simulink model "LinearInvertedPendulum_closedloop_mc40"  (R2023a)
settings: Solver=FixedStepAuto  StartTime=0.0  StopTime=inf  FixedStep=0.01  RelTol=1e-3  EnableMultiTasking=on
PreLoadFcn:
  | robotParameters;
model workspace (MAT data in the model file):
  axleLength = 0.085
  ticksPerRot = 1200
  wheelR = 0.045
undefined symbols (not defined in the file): DiscIntNeverNeededParam
libraries: M5Core_Library x4, simulink x2, arduinolib x1
settings Model: ExtModeTrigDuration=2  Creator=sseshadr  LastModifiedBy=auw_a
settings SolverCC: AlgebraicLoopSolver=TrustRegion
settings DataIOCC: ReturnWorkspaceOutputs=off
settings OptimizationCC: MaxStackSize=64  EfficientTunableParamExpr=on
settings DebuggingCC: ParameterOverflowMsg=none  ParameterUnderflowMsg=error  ParameterPrecisionLossMsg=none  ParameterTunabilityLossMsg=error  UnconnectedInputMsg=warning  UnconnectedOutputMsg=warning  UnconnectedLineMsg=warning  ArithmeticOperatorsInVariantConditions=warning
settings HardwareCC: ProdBitPerPointer=32  ProdBitPerSizeT=32  ProdBitPerPtrDiffT=32  ProdLargestAtomicInteger=Long  ProdLargestAtomicFloat=Double  ProdWordSize=32  ProdHWDeviceType=ARM Compatible->ARM Cortex
settings ModelReferenceCC: EnableRefExpFcnMdlSchedulingChecks=on
settings SFSimCC: SimUseLocalCustomCode=off  MATLABDynamicMemAlloc=off  CustomCodeUndefinedFunction=UseInterfaceOnly
settings RTWCC: Description=Embedded Coder  SystemTargetFile=ert.tlc  HardwareBoard=ESP32-WROOM(Arduino Compatible)  TLCOptions="-aInlineSetEventsForThisBaseRateFcn=TLC_FALSE -aSuppressMultiTaskScheduler=TLC_FALSE    -aRateBasedStepFcn=0"  TemplateMakefile=ert_default_tmf  GenerateReport=on  RTWUseLocalCustomCode=off  Toolchain=ESP32  BuildConfiguration=Faster Runs  IncludeHyperlinkInReport=on  GenerateTraceInfo=on  GenerateTraceReport=on  GenerateTraceReportSl=on  GenerateTraceReportSf=on  GenerateTraceReportEml=on  DLArmComputeVersion=19.05
settings CodeAppCC: ForceParamTrailComments=on  IgnoreCustomStorageClasses=off  OperatorAnnotations=on  SimulinkDataObjDesc=on  SFDataObjDesc=on  MATLABFcnDesc=on  InsertBlockDesc=on  StateflowObjectComments=on  MATLABSourceComments=on
settings ERTTargetCC: MultiwordLength=2048  SupportContinuousTime=on  SupportVariableSizeSignals=on  ExtModeTransport=3  ExtModeStaticAlloc=on  ExtModeAutomaticAllocSize=off  ExtModeStaticAllocSize=65536  ExtModeMexFile=ext_xcp  ExtModeIntrfLevel=Level2 - Open

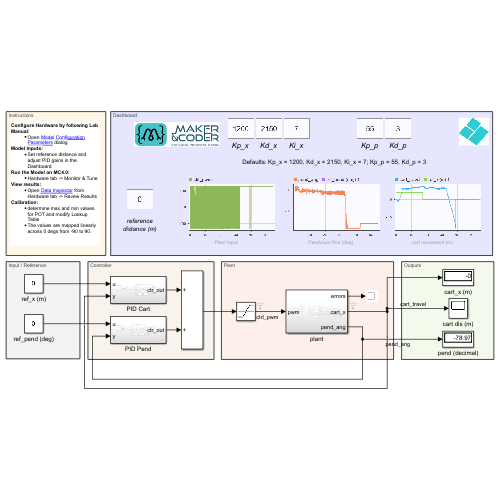
[thumbnail: Simulink's stored preview of the top-level diagram]
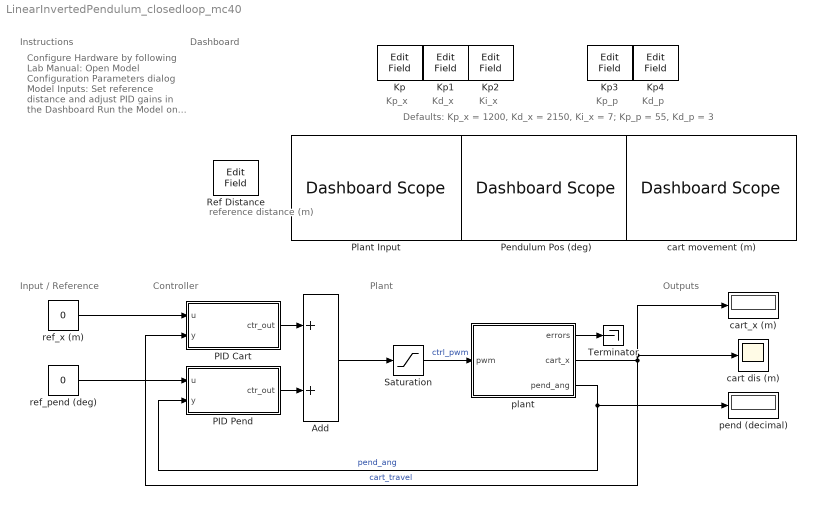
== system LinearInvertedPendulum_closedloop_mc40 ==
  note: Defaults: Kp_x = 1200, Kd_x = 2150, Ki_x = 7; Kp_p = 55, Kd_p = 3
  note: Kp_x
  note: reference
      | distance (m)
  note: Dashboard
  note: Outputs
  note: Plant
  note: Controller
  note: Input / Reference
  note: Kd_x
  note: Ki_x
  note: Configure Hardware by following Lab Manual:
      | Open Model Configuration Parameters dialog
      | Model Inputs:
      | Set reference distance and adjust PID gains in the Dashboard
      | Run the Model on MC4.0:
      | Hardware tab -> Monitor & Tune
      | View results:
      | Open Data Inspector from Hardware tab -> Revew Results
      | Calibration:
      | determine max and min values for POT and modify Lookup Table
      | The values are mapped linearly across 0 degs from -90 to 90.
  note: Instructions
  note: Kp_p
  note: Kd_p
  Add : Sum
  Kp{,1..4} (5 alike) : EditField  LabelPosition=Hide  ShowInitialText=on  Alignment=Center
  PID Cart : Subsystem
  PID Pend : Subsystem
  Pendulum Pos (deg) : DashboardScope  Ymin=-5  Ymax=5  UpdateMode=Scroll
  Plant Input : DashboardScope  Ymin=-5  Ymax=5  UpdateMode=Scroll
  Ref Distance : EditField  LabelPosition=Hide  ShowInitialText=on  Alignment=Center
  Saturation : Saturate  UpperLimit=127  LowerLimit=-127
  Terminator : Terminator
  cart dis (m) : Scope
  cart movement (m) : DashboardScope  Ymin=-5  Ymax=5  UpdateMode=Scroll
  cart_x (m) : Display
  pend (decimal) : Display
  plant : Subsystem
  ref_pend (deg) : Constant  Value=0
  ref_x (m) : Constant  Value=0
  wires:
  Saturation/1 -> plant/1(pwm)  "ctrl_pwm"
  plant/2(cart_x) -> cart_x (m)/1, cart dis (m)/1, PID Cart/2(y)  "cart_travel"
  ref_x (m)/1 -> PID Cart/1(u)
  plant/1(errors) -> Terminator/1
  PID Pend/1(ctr_out) -> Add/2
  PID Cart/1(ctr_out) -> Add/1
  Add/1 -> Saturation/1
  ref_pend (deg)/1 -> PID Pend/1(u)
  plant/3(pend_ang) -> PID Pend/2(y), pend (decimal)/1  "pend_ang"

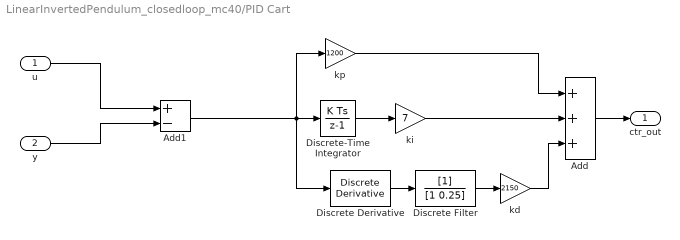
== system LinearInvertedPendulum_closedloop_mc40/PID Cart ==
  u : Inport
  y : Inport  Port=2
  Add : Sum  Inputs=+++
  Add1 : Sum  Inputs=+-
  Discrete Derivative : simulink/Discrete/Discrete Derivative  gainval=1.0  ICPrevScaledInput=0.0  OutMin=[]  OutMax=[]  OutDataType=fixdt(1, 16)  OutScaling=2^-10  DoSatur=off
  Discrete Filter : DiscreteFilter  Denominator=[1 0.25]
  Discrete-Time Integrator : DiscreteIntegrator  SampleTime=-1  ICPrevOutput=DiscIntNeverNeededParam  ICPrevScaledInput=DiscIntNeverNeededParam
  kd : Gain  Gain=2150
  ki : Gain  Gain=7
  kp : Gain  Gain=1200
  ctr_out : Outport
  wires:
  kp/1 -> Add/1
  kd/1 -> Add/3
  Discrete-Time Integrator/1 -> ki/1
  Add1/1 -> Discrete Derivative/1, Discrete-Time Integrator/1, kp/1
  Discrete Derivative/1 -> Discrete Filter/1
  ki/1 -> Add/2
  Add/1 -> ctr_out/1
  u/1 -> Add1/1
  y/1 -> Add1/2
  Discrete Filter/1 -> kd/1

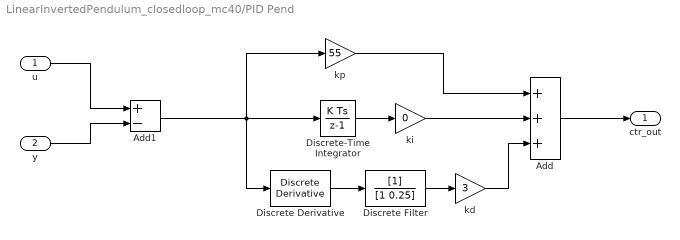
== system LinearInvertedPendulum_closedloop_mc40/PID Pend ==
  u : Inport
  y : Inport  Port=2
  Add : Sum  Inputs=+++
  Add1 : Sum  Inputs=+-
  Discrete Derivative : simulink/Discrete/Discrete Derivative  gainval=1.0  ICPrevScaledInput=0.0  OutMin=[]  OutMax=[]  OutDataType=fixdt(1, 16)  OutScaling=2^-10  DoSatur=off
  Discrete Filter : DiscreteFilter  Denominator=[1 0.25]
  Discrete-Time Integrator : DiscreteIntegrator  SampleTime=-1  ICPrevOutput=DiscIntNeverNeededParam  ICPrevScaledInput=DiscIntNeverNeededParam
  kd : Gain  Gain=3
  ki : Gain  Gain=0
  kp : Gain  Gain=55
  ctr_out : Outport
  wires:
  y/1 -> Add1/2
  u/1 -> Add1/1
  Add/1 -> ctr_out/1
  ki/1 -> Add/2
  Discrete Derivative/1 -> Discrete Filter/1
  Add1/1 -> Discrete-Time Integrator/1, kp/1, Discrete Derivative/1
  Discrete-Time Integrator/1 -> ki/1
  kd/1 -> Add/3
  kp/1 -> Add/1
  Discrete Filter/1 -> kd/1

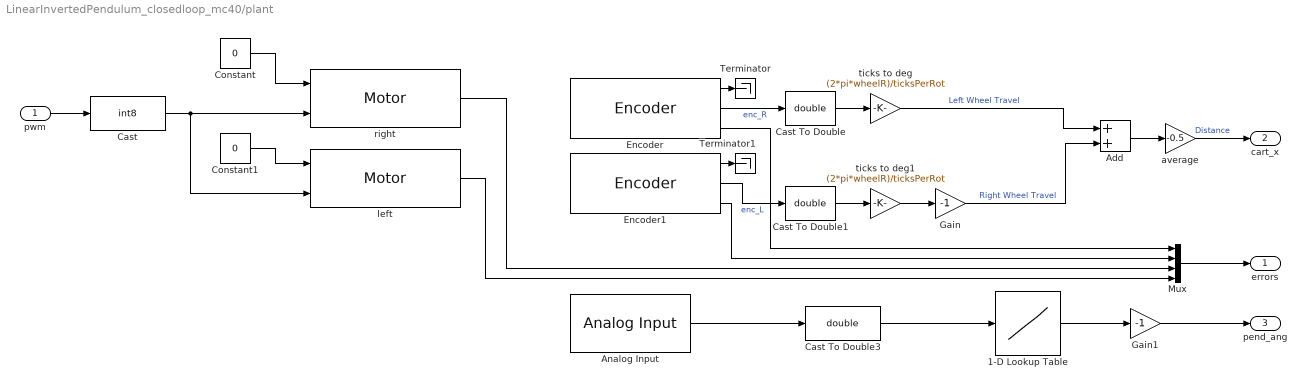
== system LinearInvertedPendulum_closedloop_mc40/plant ==
  pwm : Inport
  1-D Lookup Table : Lookup_n-D  NumberOfTableDimensions=1  BreakpointsForDimension1=linspace(2071,4095,180)  Table=linspace(90,-90,180)  ExtrapMethod=Clip  InternalRulePriority=Speed  RndMeth=Simplest
  Add : Sum
  Analog Input : arduinolib/Analog Input  pinNumber=26  ReadResultsOnly=off  ConversionTriggerSource=Software  ExternalTriggerType=uint32( 0 )  OutputDataType=uint16  EnableConversionCompleteNotify=off  EnableOuputStatus=off  SampleTime=0.01  blockPlatform=arduino
  Cast : DataTypeConversion  OutDataTypeStr=int8  SaturateOnIntegerOverflow=off  RndMeth=Floor
  Cast To Double : DataTypeConversion  OutDataTypeStr=double  SaturateOnIntegerOverflow=off  RndMeth=Floor
  Cast To Double1 : DataTypeConversion  OutDataTypeStr=double  SaturateOnIntegerOverflow=off  RndMeth=Floor
  Cast To Double3 : DataTypeConversion  OutDataTypeStr=double  SaturateOnIntegerOverflow=off  RndMeth=Floor
  Constant : Constant  Value=0
  Constant1 : Constant  Value=0
  Encoder : M5Core_Library/Encoder  M5_motor=2  s=0.01
      link override encoder I2C Read: RegisterAddress=uint8(hex2dec('40')) + m  SlaveDataType=int8
  Encoder1 : M5Core_Library/Encoder  M5_motor=1  s=0.01
  Gain : Gain  Gain=-1
  Gain1 : Gain  Gain=-1
  Mux : Mux
  Terminator : Terminator
  Terminator1 : Terminator
  average : Gain  Gain=-0.5
  left : M5Core_Library/Motor  M5_motor=M1
  right : M5Core_Library/Motor  M5_motor=M2
  ticks to deg : Gain  Gain=(2*pi*wheelR)/ticksPerRot
  ticks to deg1 : Gain  Gain=(2*pi*wheelR)/ticksPerRot
  errors : Outport
  cart_x : Outport  Port=2
  pend_ang : Outport  Port=3
  wires:
  Mux/1 -> errors/1
  Encoder/2 -> Cast To Double/1  "enc_R"
  Constant/1 -> right/1
  Constant1/1 -> left/1
  pwm/1 -> Cast/1
  average/1 -> cart_x/1  "Distance"
  Add/1 -> average/1
  ticks to deg/1 -> Add/1  "Left Wheel Travel"
  ticks to deg1/1 -> Gain/1
  Encoder1/2 -> Cast To Double1/1  "enc_L"
  Encoder/3 -> Mux/1
  Encoder1/3 -> Mux/2
  right/1 -> Mux/3
  left/1 -> Mux/4
  Encoder/1 -> Terminator/1
  Encoder1/1 -> Terminator1/1
  Gain/1 -> Add/2  "Right Wheel Travel"
  Cast To Double/1 -> ticks to deg/1
  Cast To Double1/1 -> ticks to deg1/1
  Cast/1 -> right/2, left/2
  Cast To Double3/1 -> 1-D Lookup Table/1
  1-D Lookup Table/1 -> Gain1/1
  Analog Input/1 -> Cast To Double3/1
  Gain1/1 -> pend_ang/1
